simulink model "TST_AFST_DD"  (R2016b)
settings: Solver=FixedStepDiscrete  StartTime=0.0  StopTime=simTime  FixedStep=sampleTime  RelTol=1e-3
values from neighbouring files (symbols this model uses):
  testCase = 1    [initTST_AFST_DD_001.m]    (also in initTST_AFST_DD_002.m = 2; initTST_AFST_DD_003.m = 3; initTST_AFST_DD_004.m = 4)
libraries: simulink x61, UnitTest_Lib x56
(part 1 of 2)
settings Model: Creator=guanxiaoxing  LastModifiedBy=guanxiaoxing
settings DebuggingCC: SignalRangeChecking=error

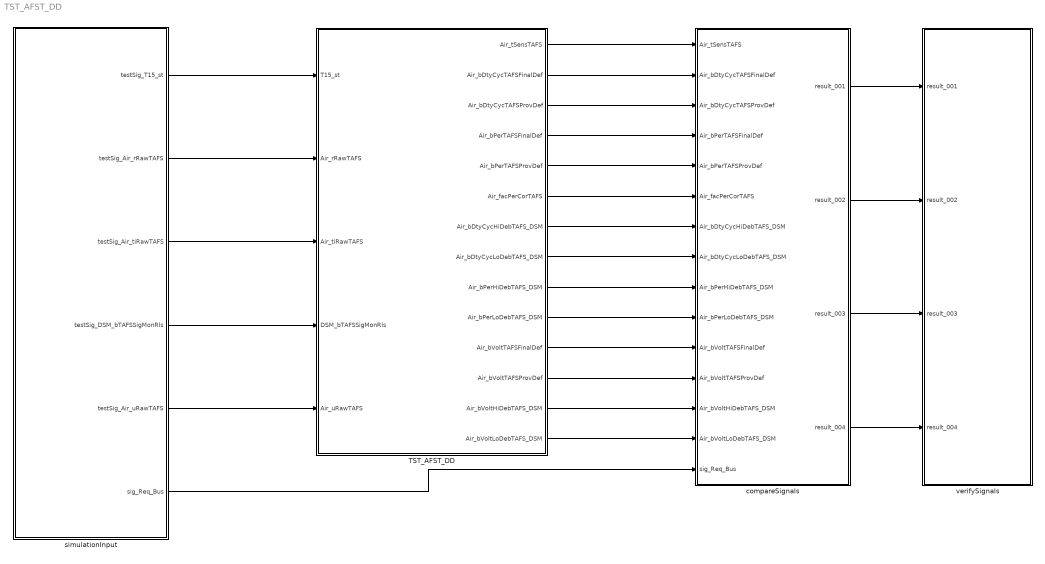
== system TST_AFST_DD ==
  TST_AFST_DD : Subsystem
  compareSignals : Subsystem
  simulationInput : Subsystem
  verifySignals : Subsystem
  wires:
  simulationInput/1(testSig_T15_st) -> TST_AFST_DD/1(T15_st)
  simulationInput/2(testSig_Air_rRawTAFS) -> TST_AFST_DD/2(Air_rRawTAFS)
  simulationInput/3(testSig_Air_tiRawTAFS) -> TST_AFST_DD/3(Air_tiRawTAFS)
  simulationInput/4(testSig_DSM_bTAFSSigMonRls) -> TST_AFST_DD/4(DSM_bTAFSSigMonRls)
  simulationInput/5(testSig_Air_uRawTAFS) -> TST_AFST_DD/5(Air_uRawTAFS)
  TST_AFST_DD/1(Air_tSensTAFS) -> compareSignals/1(Air_tSensTAFS)
  TST_AFST_DD/2(Air_bDtyCycTAFSFinalDef) -> compareSignals/2(Air_bDtyCycTAFSFinalDef)
  TST_AFST_DD/3(Air_bDtyCycTAFSProvDef) -> compareSignals/3(Air_bDtyCycTAFSProvDef)
  TST_AFST_DD/4(Air_bPerTAFSFinalDef) -> compareSignals/4(Air_bPerTAFSFinalDef)
  TST_AFST_DD/5(Air_bPerTAFSProvDef) -> compareSignals/5(Air_bPerTAFSProvDef)
  TST_AFST_DD/6(Air_facPerCorTAFS) -> compareSignals/6(Air_facPerCorTAFS)
  TST_AFST_DD/7(Air_bDtyCycHiDebTAFS_DSM) -> compareSignals/7(Air_bDtyCycHiDebTAFS_DSM)
  TST_AFST_DD/8(Air_bDtyCycLoDebTAFS_DSM) -> compareSignals/8(Air_bDtyCycLoDebTAFS_DSM)
  TST_AFST_DD/9(Air_bPerHiDebTAFS_DSM) -> compareSignals/9(Air_bPerHiDebTAFS_DSM)
  TST_AFST_DD/10(Air_bPerLoDebTAFS_DSM) -> compareSignals/10(Air_bPerLoDebTAFS_DSM)
  TST_AFST_DD/11(Air_bVoltTAFSFinalDef) -> compareSignals/11(Air_bVoltTAFSFinalDef)
  TST_AFST_DD/12(Air_bVoltTAFSProvDef) -> compareSignals/12(Air_bVoltTAFSProvDef)
  TST_AFST_DD/13(Air_bVoltHiDebTAFS_DSM) -> compareSignals/13(Air_bVoltHiDebTAFS_DSM)
  TST_AFST_DD/14(Air_bVoltLoDebTAFS_DSM) -> compareSignals/14(Air_bVoltLoDebTAFS_DSM)
  simulationInput/6(sig_Req_Bus) -> compareSignals/15(sig_Req_Bus)
  compareSignals/1(result_001) -> verifySignals/1(result_001)
  compareSignals/2(result_002) -> verifySignals/2(result_002)
  compareSignals/3(result_003) -> verifySignals/3(result_003)
  compareSignals/4(result_004) -> verifySignals/4(result_004)

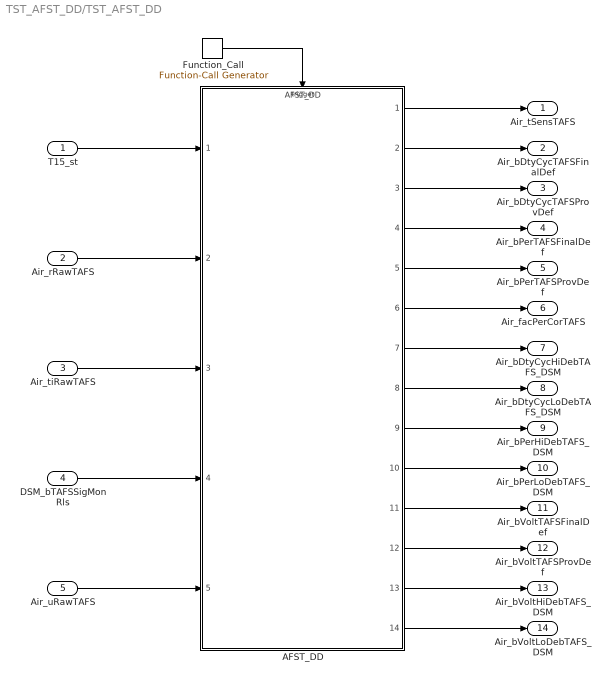
== system TST_AFST_DD/TST_AFST_DD ==
  T15_st : Inport
  Air_rRawTAFS : Inport  Port=2
  Air_tiRawTAFS : Inport  Port=3
  DSM_bTAFSSigMonRls : Inport  Port=4
  Air_uRawTAFS : Inport  Port=5
  AFST_DD : ModelReference  ModelNameDialog=AFST_DD  SimulationMode=Normal  ModelReferenceVersion=1.44  TriggerPortName=function  TriggerPortTriggerType=function-call  TriggerPortStatesWhenEnabling=held
  Function_Call : simulink/Ports & Subsystems/Function-Call Generator  sample_time=sampleTime  numberOfIterations=1
  Air_tSensTAFS : Outport
  Air_bDtyCycTAFSFinalDef : Outport  Port=2
  Air_bDtyCycTAFSProvDef : Outport  Port=3
  Air_bPerTAFSFinalDef : Outport  Port=4
  Air_bPerTAFSProvDef : Outport  Port=5
  Air_facPerCorTAFS : Outport  Port=6
  Air_bDtyCycHiDebTAFS_DSM : Outport  Port=7
  Air_bDtyCycLoDebTAFS_DSM : Outport  Port=8
  Air_bPerHiDebTAFS_DSM : Outport  Port=9
  Air_bPerLoDebTAFS_DSM : Outport  Port=10
  Air_bVoltTAFSFinalDef : Outport  Port=11
  Air_bVoltTAFSProvDef : Outport  Port=12
  Air_bVoltHiDebTAFS_DSM : Outport  Port=13
  Air_bVoltLoDebTAFS_DSM : Outport  Port=14
  wires:
  Function_Call/1 -> AFST_DD/Trigger
  T15_st/1 -> AFST_DD/1
  Air_rRawTAFS/1 -> AFST_DD/2
  Air_tiRawTAFS/1 -> AFST_DD/3
  DSM_bTAFSSigMonRls/1 -> AFST_DD/4
  Air_uRawTAFS/1 -> AFST_DD/5
  AFST_DD/1 -> Air_tSensTAFS/1
  AFST_DD/2 -> Air_bDtyCycTAFSFinalDef/1
  AFST_DD/3 -> Air_bDtyCycTAFSProvDef/1
  AFST_DD/4 -> Air_bPerTAFSFinalDef/1
  AFST_DD/5 -> Air_bPerTAFSProvDef/1
  AFST_DD/6 -> Air_facPerCorTAFS/1
  AFST_DD/7 -> Air_bDtyCycHiDebTAFS_DSM/1
  AFST_DD/8 -> Air_bDtyCycLoDebTAFS_DSM/1
  AFST_DD/9 -> Air_bPerHiDebTAFS_DSM/1
  AFST_DD/10 -> Air_bPerLoDebTAFS_DSM/1
  AFST_DD/11 -> Air_bVoltTAFSFinalDef/1
  AFST_DD/12 -> Air_bVoltTAFSProvDef/1
  AFST_DD/13 -> Air_bVoltHiDebTAFS_DSM/1
  AFST_DD/14 -> Air_bVoltLoDebTAFS_DSM/1

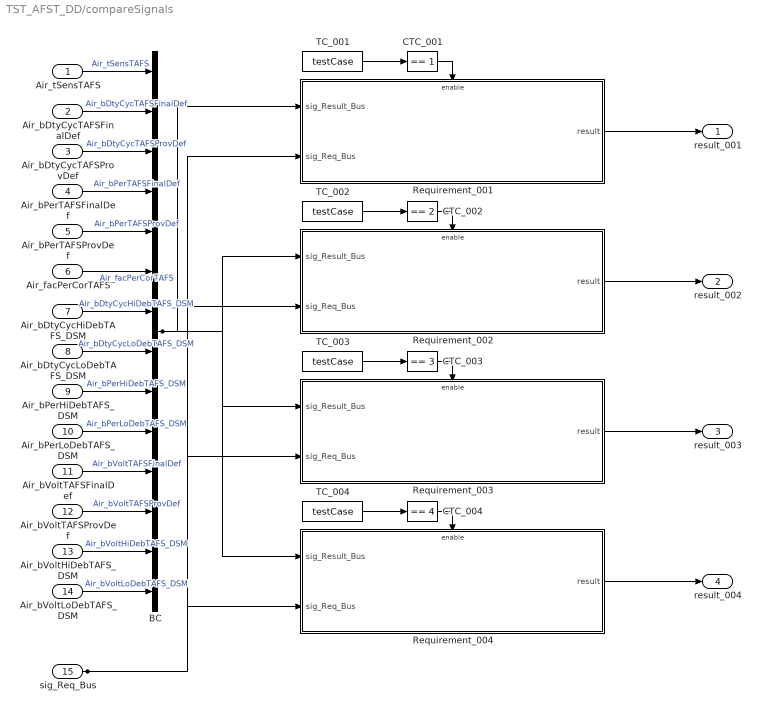
== system TST_AFST_DD/compareSignals ==
  Air_tSensTAFS : Inport
  Air_bDtyCycTAFSFinalDef : Inport  Port=2
  Air_bDtyCycTAFSProvDef : Inport  Port=3
  Air_bPerTAFSFinalDef : Inport  Port=4
  Air_bPerTAFSProvDef : Inport  Port=5
  Air_facPerCorTAFS : Inport  Port=6
  Air_bDtyCycHiDebTAFS_DSM : Inport  Port=7
  Air_bDtyCycLoDebTAFS_DSM : Inport  Port=8
  Air_bPerHiDebTAFS_DSM : Inport  Port=9
  Air_bPerLoDebTAFS_DSM : Inport  Port=10
  Air_bVoltTAFSFinalDef : Inport  Port=11
  Air_bVoltTAFSProvDef : Inport  Port=12
  Air_bVoltHiDebTAFS_DSM : Inport  Port=13
  Air_bVoltLoDebTAFS_DSM : Inport  Port=14
  sig_Req_Bus : Inport  Port=15
  BC : BusCreator  Inputs=14
  CTC_001 : simulink/Logic and Bit Operations/Compare To Constant  relop===  const=1  OutDataTypeStr=boolean
  CTC_002 : simulink/Logic and Bit Operations/Compare To Constant  relop===  const=2  OutDataTypeStr=boolean
  CTC_003 : simulink/Logic and Bit Operations/Compare To Constant  relop===  const=3  OutDataTypeStr=boolean
  CTC_004 : simulink/Logic and Bit Operations/Compare To Constant  relop===  const=4  OutDataTypeStr=boolean
  Requirement_001 : Subsystem
  Requirement_002 : Subsystem
  Requirement_003 : Subsystem
  Requirement_004 : Subsystem
  TC_001 : Constant  Value=testCase
  TC_002 : Constant  Value=testCase
  TC_003 : Constant  Value=testCase
  TC_004 : Constant  Value=testCase
  result_001 : Outport
  result_002 : Outport  Port=2
  result_003 : Outport  Port=3
  result_004 : Outport  Port=4
  wires:
  Air_tSensTAFS/1 -> BC/1  "Air_tSensTAFS"
  Air_bDtyCycTAFSFinalDef/1 -> BC/2  "Air_bDtyCycTAFSFinalDef"
  Air_bDtyCycTAFSProvDef/1 -> BC/3  "Air_bDtyCycTAFSProvDef"
  Air_bPerTAFSFinalDef/1 -> BC/4  "Air_bPerTAFSFinalDef"
  Air_bPerTAFSProvDef/1 -> BC/5  "Air_bPerTAFSProvDef"
  Air_facPerCorTAFS/1 -> BC/6  "Air_facPerCorTAFS"
  Air_bDtyCycHiDebTAFS_DSM/1 -> BC/7  "Air_bDtyCycHiDebTAFS_DSM"
  Air_bDtyCycLoDebTAFS_DSM/1 -> BC/8  "Air_bDtyCycLoDebTAFS_DSM"
  Air_bPerHiDebTAFS_DSM/1 -> BC/9  "Air_bPerHiDebTAFS_DSM"
  Air_bPerLoDebTAFS_DSM/1 -> BC/10  "Air_bPerLoDebTAFS_DSM"
  Air_bVoltTAFSFinalDef/1 -> BC/11  "Air_bVoltTAFSFinalDef"
  Air_bVoltTAFSProvDef/1 -> BC/12  "Air_bVoltTAFSProvDef"
  Air_bVoltHiDebTAFS_DSM/1 -> BC/13  "Air_bVoltHiDebTAFS_DSM"
  Air_bVoltLoDebTAFS_DSM/1 -> BC/14  "Air_bVoltLoDebTAFS_DSM"
  TC_001/1 -> CTC_001/1
  CTC_001/1 -> Requirement_001/Enable
  sig_Req_Bus/1 -> Requirement_001/2(sig_Req_Bus), Requirement_002/2(sig_Req_Bus), Requirement_003/2(sig_Req_Bus), Requirement_004/2(sig_Req_Bus)
  BC/1 -> Requirement_001/1(sig_Result_Bus), Requirement_002/1(sig_Result_Bus), Requirement_003/1(sig_Result_Bus), Requirement_004/1(sig_Result_Bus)
  Requirement_001/1(result) -> result_001/1
  TC_002/1 -> CTC_002/1
  CTC_002/1 -> Requirement_002/Enable
  Requirement_002/1(result) -> result_002/1
  TC_003/1 -> CTC_003/1
  CTC_003/1 -> Requirement_003/Enable
  Requirement_003/1(result) -> result_003/1
  TC_004/1 -> CTC_004/1
  CTC_004/1 -> Requirement_004/Enable
  Requirement_004/1(result) -> result_004/1

== system TST_AFST_DD/simulationInput ==
  BS : BusSelector  OutputSignals=testSig_T15_st,testSig_Air_rRawTAFS,testSig_Air_tiRawTAFS,testSig_DSM_bTAFSSigMonRls,testSig_Air_uRawTAFS
  MPSw : MultiPortSwitch  Inputs=4  SaturateOnIntegerOverflow=on  InputSameDT=on
  TestCase : Constant  Value=testCase
  testSignals_R001 : Subsystem
  testSignals_R002 : Subsystem
  testSignals_R003 : Subsystem
  testSignals_R004 : Subsystem
  testSig_T15_st : Outport
  testSig_Air_rRawTAFS : Outport  Port=2
  testSig_Air_tiRawTAFS : Outport  Port=3
  testSig_DSM_bTAFSSigMonRls : Outport  Port=4
  testSig_Air_uRawTAFS : Outport  Port=5
  sig_Req_Bus : Outport  Port=6
  wires:
  BS/1 -> testSig_T15_st/1  "<testSig_T15_st>"
  BS/2 -> testSig_Air_rRawTAFS/1  "<testSig_Air_rRawTAFS>"
  BS/3 -> testSig_Air_tiRawTAFS/1  "<testSig_Air_tiRawTAFS>"
  BS/4 -> testSig_DSM_bTAFSSigMonRls/1  "<testSig_DSM_bTAFSSigMonRls>"
  BS/5 -> testSig_Air_uRawTAFS/1  "<testSig_Air_uRawTAFS>"
  MPSw/1 -> BS/1, sig_Req_Bus/1
  TestCase/1 -> MPSw/1
  testSignals_R001/1(testSignals) -> MPSw/2
  testSignals_R002/1(testSignals) -> MPSw/3
  testSignals_R003/1(testSignals) -> MPSw/4
  testSignals_R004/1(testSignals) -> MPSw/5

== system TST_AFST_DD/verifySignals ==
  result_001 : Inport
  result_002 : Inport  Port=2
  result_003 : Inport  Port=3
  result_004 : Inport  Port=4
  Assertion_001 : Assertion  Enabled=off
  Assertion_002 : Assertion  Enabled=off
  Assertion_003 : Assertion  Enabled=off
  Assertion_004 : Assertion  Enabled=off
  wires:
  result_001/1 -> Assertion_001/1
  result_002/1 -> Assertion_002/1
  result_003/1 -> Assertion_003/1
  result_004/1 -> Assertion_004/1

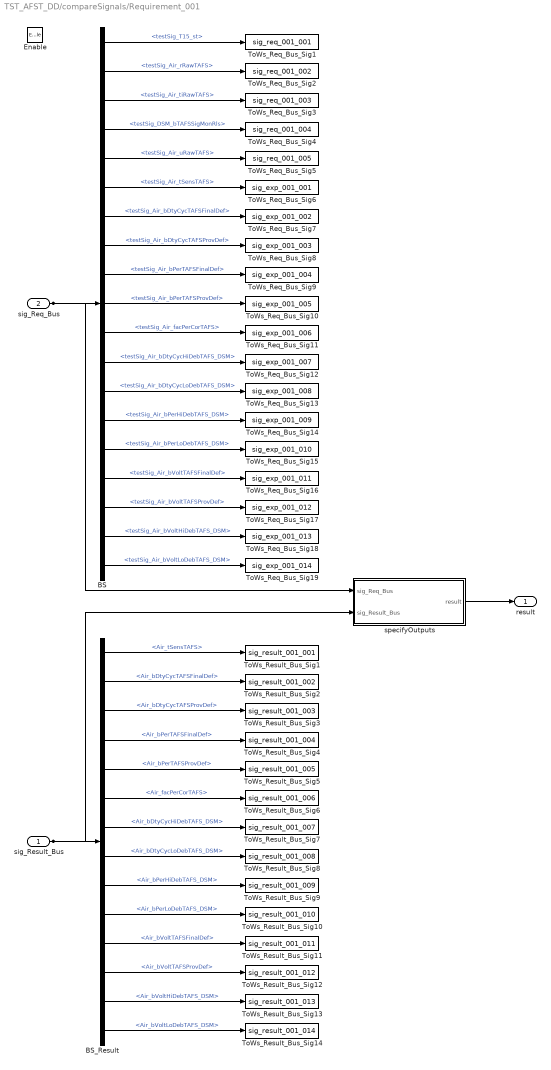
== system TST_AFST_DD/compareSignals/Requirement_001 ==
  sig_Result_Bus : Inport
  sig_Req_Bus : Inport  Port=2
  Enable : EnablePort
  BS : BusSelector  OutputSignals=testSig_T15_st,testSig_Air_rRawTAFS,testSig_Air_tiRawTAFS,testSig_DSM_bTAFSSigMonRls,testSig_Air_uRawTAFS,testSig_Air_tSensTAFS,testSig_Air_bDtyCycTAFSFinalDef,testSig_Air_bDtyCycTAFSProvDef,testSig_Air_bPerTAFSFinalDef,testSig_Air_bPerTAFSProvDef,testSig_Air_facPerCorTAFS,testSig_Air_bDtyCycHiDebTAFS_DSM,testSig_Air_bDtyCycLoDebTAFS_DSM,testSig_Air_bPerHiDebTAFS_DSM,testSig_Air_bPerLoDebTAFS_DSM,testSig_Air_bVoltTAFSFinalDef,testSig_Air_bVoltTAFSProvDef,testSig_Air_bVoltHiDebTAFS_DSM,testSig_Air_bVoltLoDebTAFS_DSM
  BS_Result : BusSelector  OutputSignals=Air_tSensTAFS,Air_bDtyCycTAFSFinalDef,Air_bDtyCycTAFSProvDef,Air_bPerTAFSFinalDef,Air_bPerTAFSProvDef,Air_facPerCorTAFS,Air_bDtyCycHiDebTAFS_DSM,Air_bDtyCycLoDebTAFS_DSM,Air_bPerHiDebTAFS_DSM,Air_bPerLoDebTAFS_DSM,Air_bVoltTAFSFinalDef,Air_bVoltTAFSProvDef,Air_bVoltHiDebTAFS_DSM,Air_bVoltLoDebTAFS_DSM
  ToWs_Req_Bus_Sig1 : ToWorkspace  VariableName=sig_req_001_001  SaveFormat=Structure With Time
  ToWs_Req_Bus_Sig10 : ToWorkspace  VariableName=sig_exp_001_005  SaveFormat=Structure With Time
  ToWs_Req_Bus_Sig11 : ToWorkspace  VariableName=sig_exp_001_006  SaveFormat=Structure With Time
  ToWs_Req_Bus_Sig12 : ToWorkspace  VariableName=sig_exp_001_007  SaveFormat=Structure With Time
  ToWs_Req_Bus_Sig13 : ToWorkspace  VariableName=sig_exp_001_008  SaveFormat=Structure With Time
  ToWs_Req_Bus_Sig14 : ToWorkspace  VariableName=sig_exp_001_009  SaveFormat=Structure With Time
  ToWs_Req_Bus_Sig15 : ToWorkspace  VariableName=sig_exp_001_010  SaveFormat=Structure With Time
  ToWs_Req_Bus_Sig16 : ToWorkspace  VariableName=sig_exp_001_011  SaveFormat=Structure With Time
  ToWs_Req_Bus_Sig17 : ToWorkspace  VariableName=sig_exp_001_012  SaveFormat=Structure With Time
  ToWs_Req_Bus_Sig18 : ToWorkspace  VariableName=sig_exp_001_013  SaveFormat=Structure With Time
  ToWs_Req_Bus_Sig19 : ToWorkspace  VariableName=sig_exp_001_014  SaveFormat=Structure With Time
  ToWs_Req_Bus_Sig2 : ToWorkspace  VariableName=sig_req_001_002  SaveFormat=Structure With Time
  ToWs_Req_Bus_Sig3 : ToWorkspace  VariableName=sig_req_001_003  SaveFormat=Structure With Time
  ToWs_Req_Bus_Sig4 : ToWorkspace  VariableName=sig_req_001_004  SaveFormat=Structure With Time
  ToWs_Req_Bus_Sig5 : ToWorkspace  VariableName=sig_req_001_005  SaveFormat=Structure With Time
  ToWs_Req_Bus_Sig6 : ToWorkspace  VariableName=sig_exp_001_001  SaveFormat=Structure With Time
  ToWs_Req_Bus_Sig7 : ToWorkspace  VariableName=sig_exp_001_002  SaveFormat=Structure With Time
  ToWs_Req_Bus_Sig8 : ToWorkspace  VariableName=sig_exp_001_003  SaveFormat=Structure With Time
  ToWs_Req_Bus_Sig9 : ToWorkspace  VariableName=sig_exp_001_004  SaveFormat=Structure With Time
  ToWs_Result_Bus_Sig1 : ToWorkspace  VariableName=sig_result_001_001  SaveFormat=Structure With Time
  ToWs_Result_Bus_Sig10 : ToWorkspace  VariableName=sig_result_001_010  SaveFormat=Structure With Time
  ToWs_Result_Bus_Sig11 : ToWorkspace  VariableName=sig_result_001_011  SaveFormat=Structure With Time
  ToWs_Result_Bus_Sig12 : ToWorkspace  VariableName=sig_result_001_012  SaveFormat=Structure With Time
  ToWs_Result_Bus_Sig13 : ToWorkspace  VariableName=sig_result_001_013  SaveFormat=Structure With Time
  ToWs_Result_Bus_Sig14 : ToWorkspace  VariableName=sig_result_001_014  SaveFormat=Structure With Time
  ToWs_Result_Bus_Sig2 : ToWorkspace  VariableName=sig_result_001_002  SaveFormat=Structure With Time
  ToWs_Result_Bus_Sig3 : ToWorkspace  VariableName=sig_result_001_003  SaveFormat=Structure With Time
  ToWs_Result_Bus_Sig4 : ToWorkspace  VariableName=sig_result_001_004  SaveFormat=Structure With Time
  ToWs_Result_Bus_Sig5 : ToWorkspace  VariableName=sig_result_001_005  SaveFormat=Structure With Time
  ToWs_Result_Bus_Sig6 : ToWorkspace  VariableName=sig_result_001_006  SaveFormat=Structure With Time
  ToWs_Result_Bus_Sig7 : ToWorkspace  VariableName=sig_result_001_007  SaveFormat=Structure With Time
  ToWs_Result_Bus_Sig8 : ToWorkspace  VariableName=sig_result_001_008  SaveFormat=Structure With Time
  ToWs_Result_Bus_Sig9 : ToWorkspace  VariableName=sig_result_001_009  SaveFormat=Structure With Time
  specifyOutputs : Subsystem
  result : Outport
  wires:
  sig_Req_Bus/1 -> BS/1, specifyOutputs/1(sig_Req_Bus)
  BS/1 -> ToWs_Req_Bus_Sig1/1  "<testSig_T15_st>"
  BS/2 -> ToWs_Req_Bus_Sig2/1  "<testSig_Air_rRawTAFS>"
  BS/3 -> ToWs_Req_Bus_Sig3/1  "<testSig_Air_tiRawTAFS>"
  BS/4 -> ToWs_Req_Bus_Sig4/1  "<testSig_DSM_bTAFSSigMonRls>"
  BS/5 -> ToWs_Req_Bus_Sig5/1  "<testSig_Air_uRawTAFS>"
  BS/6 -> ToWs_Req_Bus_Sig6/1  "<testSig_Air_tSensTAFS>"
  BS/7 -> ToWs_Req_Bus_Sig7/1  "<testSig_Air_bDtyCycTAFSFinalDef>"
  BS/8 -> ToWs_Req_Bus_Sig8/1  "<testSig_Air_bDtyCycTAFSProvDef>"
  BS/9 -> ToWs_Req_Bus_Sig9/1  "<testSig_Air_bPerTAFSFinalDef>"
  BS/10 -> ToWs_Req_Bus_Sig10/1  "<testSig_Air_bPerTAFSProvDef>"
  BS/11 -> ToWs_Req_Bus_Sig11/1  "<testSig_Air_facPerCorTAFS>"
  BS/12 -> ToWs_Req_Bus_Sig12/1  "<testSig_Air_bDtyCycHiDebTAFS_DSM>"
  BS/13 -> ToWs_Req_Bus_Sig13/1  "<testSig_Air_bDtyCycLoDebTAFS_DSM>"
  BS/14 -> ToWs_Req_Bus_Sig14/1  "<testSig_Air_bPerHiDebTAFS_DSM>"
  BS/15 -> ToWs_Req_Bus_Sig15/1  "<testSig_Air_bPerLoDebTAFS_DSM>"
  BS/16 -> ToWs_Req_Bus_Sig16/1  "<testSig_Air_bVoltTAFSFinalDef>"
  BS/17 -> ToWs_Req_Bus_Sig17/1  "<testSig_Air_bVoltTAFSProvDef>"
  BS/18 -> ToWs_Req_Bus_Sig18/1  "<testSig_Air_bVoltHiDebTAFS_DSM>"
  BS/19 -> ToWs_Req_Bus_Sig19/1  "<testSig_Air_bVoltLoDebTAFS_DSM>"
  sig_Result_Bus/1 -> BS_Result/1, specifyOutputs/2(sig_Result_Bus)
  BS_Result/1 -> ToWs_Result_Bus_Sig1/1  "<Air_tSensTAFS>"
  BS_Result/2 -> ToWs_Result_Bus_Sig2/1  "<Air_bDtyCycTAFSFinalDef>"
  BS_Result/3 -> ToWs_Result_Bus_Sig3/1  "<Air_bDtyCycTAFSProvDef>"
  BS_Result/4 -> ToWs_Result_Bus_Sig4/1  "<Air_bPerTAFSFinalDef>"
  BS_Result/5 -> ToWs_Result_Bus_Sig5/1  "<Air_bPerTAFSProvDef>"
  BS_Result/6 -> ToWs_Result_Bus_Sig6/1  "<Air_facPerCorTAFS>"
  BS_Result/7 -> ToWs_Result_Bus_Sig7/1  "<Air_bDtyCycHiDebTAFS_DSM>"
  BS_Result/8 -> ToWs_Result_Bus_Sig8/1  "<Air_bDtyCycLoDebTAFS_DSM>"
  BS_Result/9 -> ToWs_Result_Bus_Sig9/1  "<Air_bPerHiDebTAFS_DSM>"
  BS_Result/10 -> ToWs_Result_Bus_Sig10/1  "<Air_bPerLoDebTAFS_DSM>"
  BS_Result/11 -> ToWs_Result_Bus_Sig11/1  "<Air_bVoltTAFSFinalDef>"
  BS_Result/12 -> ToWs_Result_Bus_Sig12/1  "<Air_bVoltTAFSProvDef>"
  BS_Result/13 -> ToWs_Result_Bus_Sig13/1  "<Air_bVoltHiDebTAFS_DSM>"
  BS_Result/14 -> ToWs_Result_Bus_Sig14/1  "<Air_bVoltLoDebTAFS_DSM>"
  specifyOutputs/1(result) -> result/1

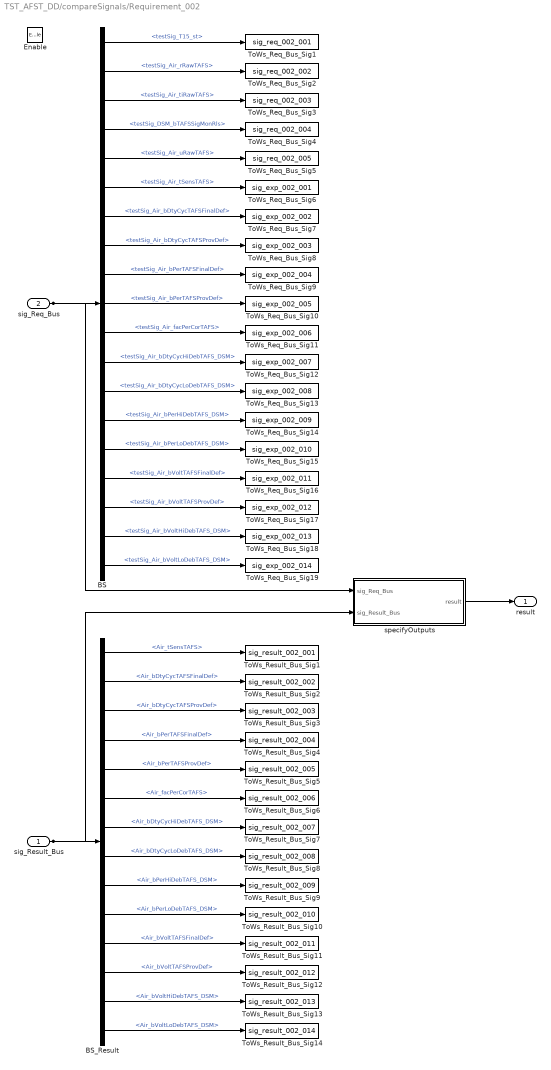
== system TST_AFST_DD/compareSignals/Requirement_002 ==
  sig_Result_Bus : Inport
  sig_Req_Bus : Inport  Port=2
  Enable : EnablePort
  BS : BusSelector  OutputSignals=testSig_T15_st,testSig_Air_rRawTAFS,testSig_Air_tiRawTAFS,testSig_DSM_bTAFSSigMonRls,testSig_Air_uRawTAFS,testSig_Air_tSensTAFS,testSig_Air_bDtyCycTAFSFinalDef,testSig_Air_bDtyCycTAFSProvDef,testSig_Air_bPerTAFSFinalDef,testSig_Air_bPerTAFSProvDef,testSig_Air_facPerCorTAFS,testSig_Air_bDtyCycHiDebTAFS_DSM,testSig_Air_bDtyCycLoDebTAFS_DSM,testSig_Air_bPerHiDebTAFS_DSM,testSig_Air_bPerLoDebTAFS_DSM,testSig_Air_bVoltTAFSFinalDef,testSig_Air_bVoltTAFSProvDef,testSig_Air_bVoltHiDebTAFS_DSM,testSig_Air_bVoltLoDebTAFS_DSM
  BS_Result : BusSelector  OutputSignals=Air_tSensTAFS,Air_bDtyCycTAFSFinalDef,Air_bDtyCycTAFSProvDef,Air_bPerTAFSFinalDef,Air_bPerTAFSProvDef,Air_facPerCorTAFS,Air_bDtyCycHiDebTAFS_DSM,Air_bDtyCycLoDebTAFS_DSM,Air_bPerHiDebTAFS_DSM,Air_bPerLoDebTAFS_DSM,Air_bVoltTAFSFinalDef,Air_bVoltTAFSProvDef,Air_bVoltHiDebTAFS_DSM,Air_bVoltLoDebTAFS_DSM
  ToWs_Req_Bus_Sig1 : ToWorkspace  VariableName=sig_req_002_001  SaveFormat=Structure With Time
  ToWs_Req_Bus_Sig10 : ToWorkspace  VariableName=sig_exp_002_005  SaveFormat=Structure With Time
  ToWs_Req_Bus_Sig11 : ToWorkspace  VariableName=sig_exp_002_006  SaveFormat=Structure With Time
  ToWs_Req_Bus_Sig12 : ToWorkspace  VariableName=sig_exp_002_007  SaveFormat=Structure With Time
  ToWs_Req_Bus_Sig13 : ToWorkspace  VariableName=sig_exp_002_008  SaveFormat=Structure With Time
  ToWs_Req_Bus_Sig14 : ToWorkspace  VariableName=sig_exp_002_009  SaveFormat=Structure With Time
  ToWs_Req_Bus_Sig15 : ToWorkspace  VariableName=sig_exp_002_010  SaveFormat=Structure With Time
  ToWs_Req_Bus_Sig16 : ToWorkspace  VariableName=sig_exp_002_011  SaveFormat=Structure With Time
  ToWs_Req_Bus_Sig17 : ToWorkspace  VariableName=sig_exp_002_012  SaveFormat=Structure With Time
  ToWs_Req_Bus_Sig18 : ToWorkspace  VariableName=sig_exp_002_013  SaveFormat=Structure With Time
  ToWs_Req_Bus_Sig19 : ToWorkspace  VariableName=sig_exp_002_014  SaveFormat=Structure With Time
  ToWs_Req_Bus_Sig2 : ToWorkspace  VariableName=sig_req_002_002  SaveFormat=Structure With Time
  ToWs_Req_Bus_Sig3 : ToWorkspace  VariableName=sig_req_002_003  SaveFormat=Structure With Time
  ToWs_Req_Bus_Sig4 : ToWorkspace  VariableName=sig_req_002_004  SaveFormat=Structure With Time
  ToWs_Req_Bus_Sig5 : ToWorkspace  VariableName=sig_req_002_005  SaveFormat=Structure With Time
  ToWs_Req_Bus_Sig6 : ToWorkspace  VariableName=sig_exp_002_001  SaveFormat=Structure With Time
  ToWs_Req_Bus_Sig7 : ToWorkspace  VariableName=sig_exp_002_002  SaveFormat=Structure With Time
  ToWs_Req_Bus_Sig8 : ToWorkspace  VariableName=sig_exp_002_003  SaveFormat=Structure With Time
  ToWs_Req_Bus_Sig9 : ToWorkspace  VariableName=sig_exp_002_004  SaveFormat=Structure With Time
  ToWs_Result_Bus_Sig1 : ToWorkspace  VariableName=sig_result_002_001  SaveFormat=Structure With Time
  ToWs_Result_Bus_Sig10 : ToWorkspace  VariableName=sig_result_002_010  SaveFormat=Structure With Time
  ToWs_Result_Bus_Sig11 : ToWorkspace  VariableName=sig_result_002_011  SaveFormat=Structure With Time
  ToWs_Result_Bus_Sig12 : ToWorkspace  VariableName=sig_result_002_012  SaveFormat=Structure With Time
  ToWs_Result_Bus_Sig13 : ToWorkspace  VariableName=sig_result_002_013  SaveFormat=Structure With Time
  ToWs_Result_Bus_Sig14 : ToWorkspace  VariableName=sig_result_002_014  SaveFormat=Structure With Time
  ToWs_Result_Bus_Sig2 : ToWorkspace  VariableName=sig_result_002_002  SaveFormat=Structure With Time
  ToWs_Result_Bus_Sig3 : ToWorkspace  VariableName=sig_result_002_003  SaveFormat=Structure With Time
  ToWs_Result_Bus_Sig4 : ToWorkspace  VariableName=sig_result_002_004  SaveFormat=Structure With Time
  ToWs_Result_Bus_Sig5 : ToWorkspace  VariableName=sig_result_002_005  SaveFormat=Structure With Time
  ToWs_Result_Bus_Sig6 : ToWorkspace  VariableName=sig_result_002_006  SaveFormat=Structure With Time
  ToWs_Result_Bus_Sig7 : ToWorkspace  VariableName=sig_result_002_007  SaveFormat=Structure With Time
  ToWs_Result_Bus_Sig8 : ToWorkspace  VariableName=sig_result_002_008  SaveFormat=Structure With Time
  ToWs_Result_Bus_Sig9 : ToWorkspace  VariableName=sig_result_002_009  SaveFormat=Structure With Time
  specifyOutputs : Subsystem
  result : Outport
  wires:
  sig_Req_Bus/1 -> BS/1, specifyOutputs/1(sig_Req_Bus)
  BS/1 -> ToWs_Req_Bus_Sig1/1  "<testSig_T15_st>"
  BS/2 -> ToWs_Req_Bus_Sig2/1  "<testSig_Air_rRawTAFS>"
  BS/3 -> ToWs_Req_Bus_Sig3/1  "<testSig_Air_tiRawTAFS>"
  BS/4 -> ToWs_Req_Bus_Sig4/1  "<testSig_DSM_bTAFSSigMonRls>"
  BS/5 -> ToWs_Req_Bus_Sig5/1  "<testSig_Air_uRawTAFS>"
  BS/6 -> ToWs_Req_Bus_Sig6/1  "<testSig_Air_tSensTAFS>"
  BS/7 -> ToWs_Req_Bus_Sig7/1  "<testSig_Air_bDtyCycTAFSFinalDef>"
  BS/8 -> ToWs_Req_Bus_Sig8/1  "<testSig_Air_bDtyCycTAFSProvDef>"
  BS/9 -> ToWs_Req_Bus_Sig9/1  "<testSig_Air_bPerTAFSFinalDef>"
  BS/10 -> ToWs_Req_Bus_Sig10/1  "<testSig_Air_bPerTAFSProvDef>"
  BS/11 -> ToWs_Req_Bus_Sig11/1  "<testSig_Air_facPerCorTAFS>"
  BS/12 -> ToWs_Req_Bus_Sig12/1  "<testSig_Air_bDtyCycHiDebTAFS_DSM>"
  BS/13 -> ToWs_Req_Bus_Sig13/1  "<testSig_Air_bDtyCycLoDebTAFS_DSM>"
  BS/14 -> ToWs_Req_Bus_Sig14/1  "<testSig_Air_bPerHiDebTAFS_DSM>"
  BS/15 -> ToWs_Req_Bus_Sig15/1  "<testSig_Air_bPerLoDebTAFS_DSM>"
  BS/16 -> ToWs_Req_Bus_Sig16/1  "<testSig_Air_bVoltTAFSFinalDef>"
  BS/17 -> ToWs_Req_Bus_Sig17/1  "<testSig_Air_bVoltTAFSProvDef>"
  BS/18 -> ToWs_Req_Bus_Sig18/1  "<testSig_Air_bVoltHiDebTAFS_DSM>"
  BS/19 -> ToWs_Req_Bus_Sig19/1  "<testSig_Air_bVoltLoDebTAFS_DSM>"
  sig_Result_Bus/1 -> BS_Result/1, specifyOutputs/2(sig_Result_Bus)
  BS_Result/1 -> ToWs_Result_Bus_Sig1/1  "<Air_tSensTAFS>"
  BS_Result/2 -> ToWs_Result_Bus_Sig2/1  "<Air_bDtyCycTAFSFinalDef>"
  BS_Result/3 -> ToWs_Result_Bus_Sig3/1  "<Air_bDtyCycTAFSProvDef>"
  BS_Result/4 -> ToWs_Result_Bus_Sig4/1  "<Air_bPerTAFSFinalDef>"
  BS_Result/5 -> ToWs_Result_Bus_Sig5/1  "<Air_bPerTAFSProvDef>"
  BS_Result/6 -> ToWs_Result_Bus_Sig6/1  "<Air_facPerCorTAFS>"
  BS_Result/7 -> ToWs_Result_Bus_Sig7/1  "<Air_bDtyCycHiDebTAFS_DSM>"
  BS_Result/8 -> ToWs_Result_Bus_Sig8/1  "<Air_bDtyCycLoDebTAFS_DSM>"
  BS_Result/9 -> ToWs_Result_Bus_Sig9/1  "<Air_bPerHiDebTAFS_DSM>"
  BS_Result/10 -> ToWs_Result_Bus_Sig10/1  "<Air_bPerLoDebTAFS_DSM>"
  BS_Result/11 -> ToWs_Result_Bus_Sig11/1  "<Air_bVoltTAFSFinalDef>"
  BS_Result/12 -> ToWs_Result_Bus_Sig12/1  "<Air_bVoltTAFSProvDef>"
  BS_Result/13 -> ToWs_Result_Bus_Sig13/1  "<Air_bVoltHiDebTAFS_DSM>"
  BS_Result/14 -> ToWs_Result_Bus_Sig14/1  "<Air_bVoltLoDebTAFS_DSM>"
  specifyOutputs/1(result) -> result/1

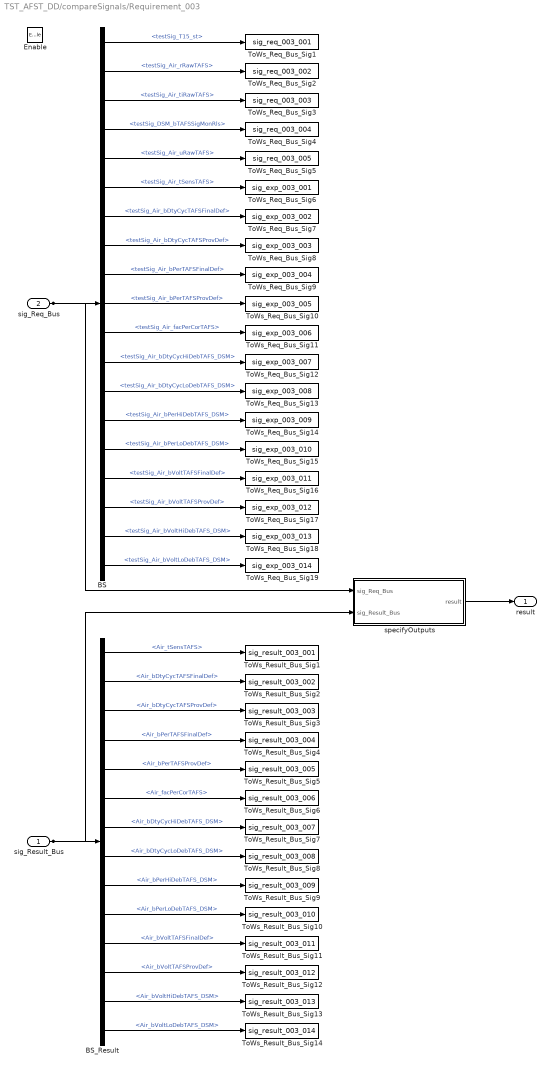
== system TST_AFST_DD/compareSignals/Requirement_003 ==
  sig_Result_Bus : Inport
  sig_Req_Bus : Inport  Port=2
  Enable : EnablePort
  BS : BusSelector  OutputSignals=testSig_T15_st,testSig_Air_rRawTAFS,testSig_Air_tiRawTAFS,testSig_DSM_bTAFSSigMonRls,testSig_Air_uRawTAFS,testSig_Air_tSensTAFS,testSig_Air_bDtyCycTAFSFinalDef,testSig_Air_bDtyCycTAFSProvDef,testSig_Air_bPerTAFSFinalDef,testSig_Air_bPerTAFSProvDef,testSig_Air_facPerCorTAFS,testSig_Air_bDtyCycHiDebTAFS_DSM,testSig_Air_bDtyCycLoDebTAFS_DSM,testSig_Air_bPerHiDebTAFS_DSM,testSig_Air_bPerLoDebTAFS_DSM,testSig_Air_bVoltTAFSFinalDef,testSig_Air_bVoltTAFSProvDef,testSig_Air_bVoltHiDebTAFS_DSM,testSig_Air_bVoltLoDebTAFS_DSM
  BS_Result : BusSelector  OutputSignals=Air_tSensTAFS,Air_bDtyCycTAFSFinalDef,Air_bDtyCycTAFSProvDef,Air_bPerTAFSFinalDef,Air_bPerTAFSProvDef,Air_facPerCorTAFS,Air_bDtyCycHiDebTAFS_DSM,Air_bDtyCycLoDebTAFS_DSM,Air_bPerHiDebTAFS_DSM,Air_bPerLoDebTAFS_DSM,Air_bVoltTAFSFinalDef,Air_bVoltTAFSProvDef,Air_bVoltHiDebTAFS_DSM,Air_bVoltLoDebTAFS_DSM
  ToWs_Req_Bus_Sig1 : ToWorkspace  VariableName=sig_req_003_001  SaveFormat=Structure With Time
  ToWs_Req_Bus_Sig10 : ToWorkspace  VariableName=sig_exp_003_005  SaveFormat=Structure With Time
  ToWs_Req_Bus_Sig11 : ToWorkspace  VariableName=sig_exp_003_006  SaveFormat=Structure With Time
  ToWs_Req_Bus_Sig12 : ToWorkspace  VariableName=sig_exp_003_007  SaveFormat=Structure With Time
  ToWs_Req_Bus_Sig13 : ToWorkspace  VariableName=sig_exp_003_008  SaveFormat=Structure With Time
  ToWs_Req_Bus_Sig14 : ToWorkspace  VariableName=sig_exp_003_009  SaveFormat=Structure With Time
  ToWs_Req_Bus_Sig15 : ToWorkspace  VariableName=sig_exp_003_010  SaveFormat=Structure With Time
  ToWs_Req_Bus_Sig16 : ToWorkspace  VariableName=sig_exp_003_011  SaveFormat=Structure With Time
  ToWs_Req_Bus_Sig17 : ToWorkspace  VariableName=sig_exp_003_012  SaveFormat=Structure With Time
  ToWs_Req_Bus_Sig18 : ToWorkspace  VariableName=sig_exp_003_013  SaveFormat=Structure With Time
  ToWs_Req_Bus_Sig19 : ToWorkspace  VariableName=sig_exp_003_014  SaveFormat=Structure With Time
  ToWs_Req_Bus_Sig2 : ToWorkspace  VariableName=sig_req_003_002  SaveFormat=Structure With Time
  ToWs_Req_Bus_Sig3 : ToWorkspace  VariableName=sig_req_003_003  SaveFormat=Structure With Time
  ToWs_Req_Bus_Sig4 : ToWorkspace  VariableName=sig_req_003_004  SaveFormat=Structure With Time
  ToWs_Req_Bus_Sig5 : ToWorkspace  VariableName=sig_req_003_005  SaveFormat=Structure With Time
  ToWs_Req_Bus_Sig6 : ToWorkspace  VariableName=sig_exp_003_001  SaveFormat=Structure With Time
  ToWs_Req_Bus_Sig7 : ToWorkspace  VariableName=sig_exp_003_002  SaveFormat=Structure With Time
  ToWs_Req_Bus_Sig8 : ToWorkspace  VariableName=sig_exp_003_003  SaveFormat=Structure With Time
  ToWs_Req_Bus_Sig9 : ToWorkspace  VariableName=sig_exp_003_004  SaveFormat=Structure With Time
  ToWs_Result_Bus_Sig1 : ToWorkspace  VariableName=sig_result_003_001  SaveFormat=Structure With Time
  ToWs_Result_Bus_Sig10 : ToWorkspace  VariableName=sig_result_003_010  SaveFormat=Structure With Time
  ToWs_Result_Bus_Sig11 : ToWorkspace  VariableName=sig_result_003_011  SaveFormat=Structure With Time
  ToWs_Result_Bus_Sig12 : ToWorkspace  VariableName=sig_result_003_012  SaveFormat=Structure With Time
  ToWs_Result_Bus_Sig13 : ToWorkspace  VariableName=sig_result_003_013  SaveFormat=Structure With Time
  ToWs_Result_Bus_Sig14 : ToWorkspace  VariableName=sig_result_003_014  SaveFormat=Structure With Time
  ToWs_Result_Bus_Sig2 : ToWorkspace  VariableName=sig_result_003_002  SaveFormat=Structure With Time
  ToWs_Result_Bus_Sig3 : ToWorkspace  VariableName=sig_result_003_003  SaveFormat=Structure With Time
  ToWs_Result_Bus_Sig4 : ToWorkspace  VariableName=sig_result_003_004  SaveFormat=Structure With Time
  ToWs_Result_Bus_Sig5 : ToWorkspace  VariableName=sig_result_003_005  SaveFormat=Structure With Time
  ToWs_Result_Bus_Sig6 : ToWorkspace  VariableName=sig_result_003_006  SaveFormat=Structure With Time
  ToWs_Result_Bus_Sig7 : ToWorkspace  VariableName=sig_result_003_007  SaveFormat=Structure With Time
  ToWs_Result_Bus_Sig8 : ToWorkspace  VariableName=sig_result_003_008  SaveFormat=Structure With Time
  ToWs_Result_Bus_Sig9 : ToWorkspace  VariableName=sig_result_003_009  SaveFormat=Structure With Time
  specifyOutputs : Subsystem
  result : Outport
  wires:
  sig_Req_Bus/1 -> BS/1, specifyOutputs/1(sig_Req_Bus)
  BS/1 -> ToWs_Req_Bus_Sig1/1  "<testSig_T15_st>"
  BS/2 -> ToWs_Req_Bus_Sig2/1  "<testSig_Air_rRawTAFS>"
  BS/3 -> ToWs_Req_Bus_Sig3/1  "<testSig_Air_tiRawTAFS>"
  BS/4 -> ToWs_Req_Bus_Sig4/1  "<testSig_DSM_bTAFSSigMonRls>"
  BS/5 -> ToWs_Req_Bus_Sig5/1  "<testSig_Air_uRawTAFS>"
  BS/6 -> ToWs_Req_Bus_Sig6/1  "<testSig_Air_tSensTAFS>"
  BS/7 -> ToWs_Req_Bus_Sig7/1  "<testSig_Air_bDtyCycTAFSFinalDef>"
  BS/8 -> ToWs_Req_Bus_Sig8/1  "<testSig_Air_bDtyCycTAFSProvDef>"
  BS/9 -> ToWs_Req_Bus_Sig9/1  "<testSig_Air_bPerTAFSFinalDef>"
  BS/10 -> ToWs_Req_Bus_Sig10/1  "<testSig_Air_bPerTAFSProvDef>"
  BS/11 -> ToWs_Req_Bus_Sig11/1  "<testSig_Air_facPerCorTAFS>"
  BS/12 -> ToWs_Req_Bus_Sig12/1  "<testSig_Air_bDtyCycHiDebTAFS_DSM>"
  BS/13 -> ToWs_Req_Bus_Sig13/1  "<testSig_Air_bDtyCycLoDebTAFS_DSM>"
  BS/14 -> ToWs_Req_Bus_Sig14/1  "<testSig_Air_bPerHiDebTAFS_DSM>"
  BS/15 -> ToWs_Req_Bus_Sig15/1  "<testSig_Air_bPerLoDebTAFS_DSM>"
  BS/16 -> ToWs_Req_Bus_Sig16/1  "<testSig_Air_bVoltTAFSFinalDef>"
  BS/17 -> ToWs_Req_Bus_Sig17/1  "<testSig_Air_bVoltTAFSProvDef>"
  BS/18 -> ToWs_Req_Bus_Sig18/1  "<testSig_Air_bVoltHiDebTAFS_DSM>"
  BS/19 -> ToWs_Req_Bus_Sig19/1  "<testSig_Air_bVoltLoDebTAFS_DSM>"
  sig_Result_Bus/1 -> BS_Result/1, specifyOutputs/2(sig_Result_Bus)
  BS_Result/1 -> ToWs_Result_Bus_Sig1/1  "<Air_tSensTAFS>"
  BS_Result/2 -> ToWs_Result_Bus_Sig2/1  "<Air_bDtyCycTAFSFinalDef>"
  BS_Result/3 -> ToWs_Result_Bus_Sig3/1  "<Air_bDtyCycTAFSProvDef>"
  BS_Result/4 -> ToWs_Result_Bus_Sig4/1  "<Air_bPerTAFSFinalDef>"
  BS_Result/5 -> ToWs_Result_Bus_Sig5/1  "<Air_bPerTAFSProvDef>"
  BS_Result/6 -> ToWs_Result_Bus_Sig6/1  "<Air_facPerCorTAFS>"
  BS_Result/7 -> ToWs_Result_Bus_Sig7/1  "<Air_bDtyCycHiDebTAFS_DSM>"
  BS_Result/8 -> ToWs_Result_Bus_Sig8/1  "<Air_bDtyCycLoDebTAFS_DSM>"
  BS_Result/9 -> ToWs_Result_Bus_Sig9/1  "<Air_bPerHiDebTAFS_DSM>"
  BS_Result/10 -> ToWs_Result_Bus_Sig10/1  "<Air_bPerLoDebTAFS_DSM>"
  BS_Result/11 -> ToWs_Result_Bus_Sig11/1  "<Air_bVoltTAFSFinalDef>"
  BS_Result/12 -> ToWs_Result_Bus_Sig12/1  "<Air_bVoltTAFSProvDef>"
  BS_Result/13 -> ToWs_Result_Bus_Sig13/1  "<Air_bVoltHiDebTAFS_DSM>"
  BS_Result/14 -> ToWs_Result_Bus_Sig14/1  "<Air_bVoltLoDebTAFS_DSM>"
  specifyOutputs/1(result) -> result/1

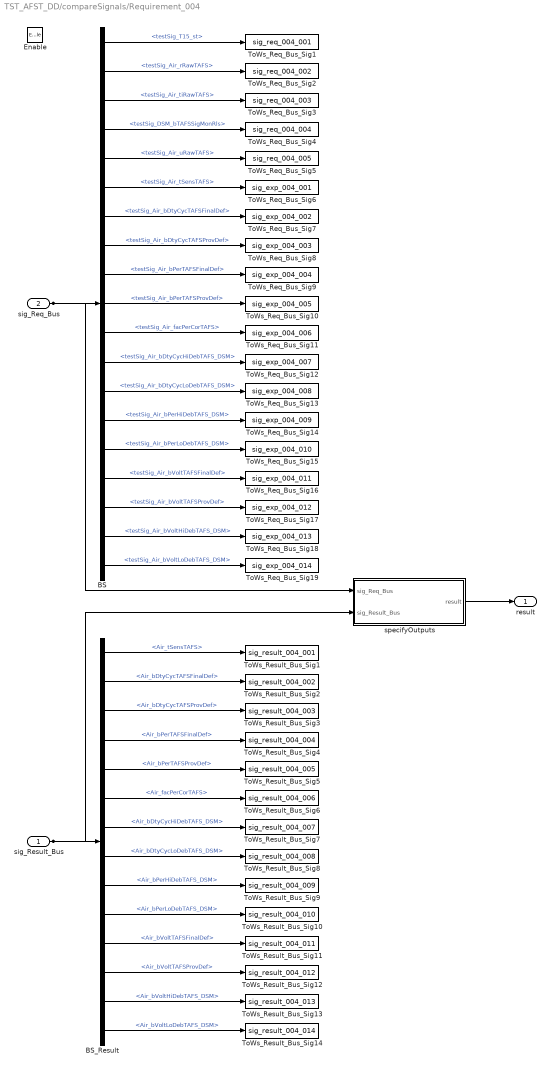
== system TST_AFST_DD/compareSignals/Requirement_004 ==
  sig_Result_Bus : Inport
  sig_Req_Bus : Inport  Port=2
  Enable : EnablePort
  BS : BusSelector  OutputSignals=testSig_T15_st,testSig_Air_rRawTAFS,testSig_Air_tiRawTAFS,testSig_DSM_bTAFSSigMonRls,testSig_Air_uRawTAFS,testSig_Air_tSensTAFS,testSig_Air_bDtyCycTAFSFinalDef,testSig_Air_bDtyCycTAFSProvDef,testSig_Air_bPerTAFSFinalDef,testSig_Air_bPerTAFSProvDef,testSig_Air_facPerCorTAFS,testSig_Air_bDtyCycHiDebTAFS_DSM,testSig_Air_bDtyCycLoDebTAFS_DSM,testSig_Air_bPerHiDebTAFS_DSM,testSig_Air_bPerLoDebTAFS_DSM,testSig_Air_bVoltTAFSFinalDef,testSig_Air_bVoltTAFSProvDef,testSig_Air_bVoltHiDebTAFS_DSM,testSig_Air_bVoltLoDebTAFS_DSM
  BS_Result : BusSelector  OutputSignals=Air_tSensTAFS,Air_bDtyCycTAFSFinalDef,Air_bDtyCycTAFSProvDef,Air_bPerTAFSFinalDef,Air_bPerTAFSProvDef,Air_facPerCorTAFS,Air_bDtyCycHiDebTAFS_DSM,Air_bDtyCycLoDebTAFS_DSM,Air_bPerHiDebTAFS_DSM,Air_bPerLoDebTAFS_DSM,Air_bVoltTAFSFinalDef,Air_bVoltTAFSProvDef,Air_bVoltHiDebTAFS_DSM,Air_bVoltLoDebTAFS_DSM
  ToWs_Req_Bus_Sig1 : ToWorkspace  VariableName=sig_req_004_001  SaveFormat=Structure With Time
  ToWs_Req_Bus_Sig10 : ToWorkspace  VariableName=sig_exp_004_005  SaveFormat=Structure With Time
  ToWs_Req_Bus_Sig11 : ToWorkspace  VariableName=sig_exp_004_006  SaveFormat=Structure With Time
  ToWs_Req_Bus_Sig12 : ToWorkspace  VariableName=sig_exp_004_007  SaveFormat=Structure With Time
  ToWs_Req_Bus_Sig13 : ToWorkspace  VariableName=sig_exp_004_008  SaveFormat=Structure With Time
  ToWs_Req_Bus_Sig14 : ToWorkspace  VariableName=sig_exp_004_009  SaveFormat=Structure With Time
  ToWs_Req_Bus_Sig15 : ToWorkspace  VariableName=sig_exp_004_010  SaveFormat=Structure With Time
  ToWs_Req_Bus_Sig16 : ToWorkspace  VariableName=sig_exp_004_011  SaveFormat=Structure With Time
  ToWs_Req_Bus_Sig17 : ToWorkspace  VariableName=sig_exp_004_012  SaveFormat=Structure With Time
  ToWs_Req_Bus_Sig18 : ToWorkspace  VariableName=sig_exp_004_013  SaveFormat=Structure With Time
  ToWs_Req_Bus_Sig19 : ToWorkspace  VariableName=sig_exp_004_014  SaveFormat=Structure With Time
  ToWs_Req_Bus_Sig2 : ToWorkspace  VariableName=sig_req_004_002  SaveFormat=Structure With Time
  ToWs_Req_Bus_Sig3 : ToWorkspace  VariableName=sig_req_004_003  SaveFormat=Structure With Time
  ToWs_Req_Bus_Sig4 : ToWorkspace  VariableName=sig_req_004_004  SaveFormat=Structure With Time
  ToWs_Req_Bus_Sig5 : ToWorkspace  VariableName=sig_req_004_005  SaveFormat=Structure With Time
  ToWs_Req_Bus_Sig6 : ToWorkspace  VariableName=sig_exp_004_001  SaveFormat=Structure With Time
  ToWs_Req_Bus_Sig7 : ToWorkspace  VariableName=sig_exp_004_002  SaveFormat=Structure With Time
  ToWs_Req_Bus_Sig8 : ToWorkspace  VariableName=sig_exp_004_003  SaveFormat=Structure With Time
  ToWs_Req_Bus_Sig9 : ToWorkspace  VariableName=sig_exp_004_004  SaveFormat=Structure With Time
  ToWs_Result_Bus_Sig1 : ToWorkspace  VariableName=sig_result_004_001  SaveFormat=Structure With Time
  ToWs_Result_Bus_Sig10 : ToWorkspace  VariableName=sig_result_004_010  SaveFormat=Structure With Time
  ToWs_Result_Bus_Sig11 : ToWorkspace  VariableName=sig_result_004_011  SaveFormat=Structure With Time
  ToWs_Result_Bus_Sig12 : ToWorkspace  VariableName=sig_result_004_012  SaveFormat=Structure With Time
  ToWs_Result_Bus_Sig13 : ToWorkspace  VariableName=sig_result_004_013  SaveFormat=Structure With Time
  ToWs_Result_Bus_Sig14 : ToWorkspace  VariableName=sig_result_004_014  SaveFormat=Structure With Time
  ToWs_Result_Bus_Sig2 : ToWorkspace  VariableName=sig_result_004_002  SaveFormat=Structure With Time
  ToWs_Result_Bus_Sig3 : ToWorkspace  VariableName=sig_result_004_003  SaveFormat=Structure With Time
  ToWs_Result_Bus_Sig4 : ToWorkspace  VariableName=sig_result_004_004  SaveFormat=Structure With Time
  ToWs_Result_Bus_Sig5 : ToWorkspace  VariableName=sig_result_004_005  SaveFormat=Structure With Time
  ToWs_Result_Bus_Sig6 : ToWorkspace  VariableName=sig_result_004_006  SaveFormat=Structure With Time
  ToWs_Result_Bus_Sig7 : ToWorkspace  VariableName=sig_result_004_007  SaveFormat=Structure With Time
  ToWs_Result_Bus_Sig8 : ToWorkspace  VariableName=sig_result_004_008  SaveFormat=Structure With Time
  ToWs_Result_Bus_Sig9 : ToWorkspace  VariableName=sig_result_004_009  SaveFormat=Structure With Time
  specifyOutputs : Subsystem
  result : Outport
  wires:
  sig_Req_Bus/1 -> BS/1, specifyOutputs/1(sig_Req_Bus)
  BS/1 -> ToWs_Req_Bus_Sig1/1  "<testSig_T15_st>"
  BS/2 -> ToWs_Req_Bus_Sig2/1  "<testSig_Air_rRawTAFS>"
  BS/3 -> ToWs_Req_Bus_Sig3/1  "<testSig_Air_tiRawTAFS>"
  BS/4 -> ToWs_Req_Bus_Sig4/1  "<testSig_DSM_bTAFSSigMonRls>"
  BS/5 -> ToWs_Req_Bus_Sig5/1  "<testSig_Air_uRawTAFS>"
  BS/6 -> ToWs_Req_Bus_Sig6/1  "<testSig_Air_tSensTAFS>"
  BS/7 -> ToWs_Req_Bus_Sig7/1  "<testSig_Air_bDtyCycTAFSFinalDef>"
  BS/8 -> ToWs_Req_Bus_Sig8/1  "<testSig_Air_bDtyCycTAFSProvDef>"
  BS/9 -> ToWs_Req_Bus_Sig9/1  "<testSig_Air_bPerTAFSFinalDef>"
  BS/10 -> ToWs_Req_Bus_Sig10/1  "<testSig_Air_bPerTAFSProvDef>"
  BS/11 -> ToWs_Req_Bus_Sig11/1  "<testSig_Air_facPerCorTAFS>"
  BS/12 -> ToWs_Req_Bus_Sig12/1  "<testSig_Air_bDtyCycHiDebTAFS_DSM>"
  BS/13 -> ToWs_Req_Bus_Sig13/1  "<testSig_Air_bDtyCycLoDebTAFS_DSM>"
  BS/14 -> ToWs_Req_Bus_Sig14/1  "<testSig_Air_bPerHiDebTAFS_DSM>"
  BS/15 -> ToWs_Req_Bus_Sig15/1  "<testSig_Air_bPerLoDebTAFS_DSM>"
  BS/16 -> ToWs_Req_Bus_Sig16/1  "<testSig_Air_bVoltTAFSFinalDef>"
  BS/17 -> ToWs_Req_Bus_Sig17/1  "<testSig_Air_bVoltTAFSProvDef>"
  BS/18 -> ToWs_Req_Bus_Sig18/1  "<testSig_Air_bVoltHiDebTAFS_DSM>"
  BS/19 -> ToWs_Req_Bus_Sig19/1  "<testSig_Air_bVoltLoDebTAFS_DSM>"
  sig_Result_Bus/1 -> BS_Result/1, specifyOutputs/2(sig_Result_Bus)
  BS_Result/1 -> ToWs_Result_Bus_Sig1/1  "<Air_tSensTAFS>"
  BS_Result/2 -> ToWs_Result_Bus_Sig2/1  "<Air_bDtyCycTAFSFinalDef>"
  BS_Result/3 -> ToWs_Result_Bus_Sig3/1  "<Air_bDtyCycTAFSProvDef>"
  BS_Result/4 -> ToWs_Result_Bus_Sig4/1  "<Air_bPerTAFSFinalDef>"
  BS_Result/5 -> ToWs_Result_Bus_Sig5/1  "<Air_bPerTAFSProvDef>"
  BS_Result/6 -> ToWs_Result_Bus_Sig6/1  "<Air_facPerCorTAFS>"
  BS_Result/7 -> ToWs_Result_Bus_Sig7/1  "<Air_bDtyCycHiDebTAFS_DSM>"
  BS_Result/8 -> ToWs_Result_Bus_Sig8/1  "<Air_bDtyCycLoDebTAFS_DSM>"
  BS_Result/9 -> ToWs_Result_Bus_Sig9/1  "<Air_bPerHiDebTAFS_DSM>"
  BS_Result/10 -> ToWs_Result_Bus_Sig10/1  "<Air_bPerLoDebTAFS_DSM>"
  BS_Result/11 -> ToWs_Result_Bus_Sig11/1  "<Air_bVoltTAFSFinalDef>"
  BS_Result/12 -> ToWs_Result_Bus_Sig12/1  "<Air_bVoltTAFSProvDef>"
  BS_Result/13 -> ToWs_Result_Bus_Sig13/1  "<Air_bVoltHiDebTAFS_DSM>"
  BS_Result/14 -> ToWs_Result_Bus_Sig14/1  "<Air_bVoltLoDebTAFS_DSM>"
  specifyOutputs/1(result) -> result/1

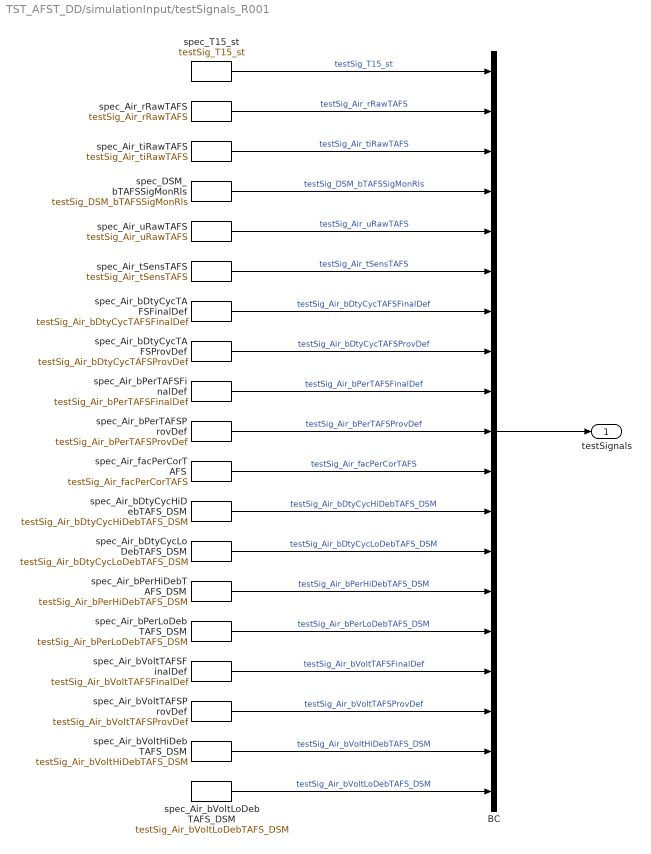
== system TST_AFST_DD/simulationInput/testSignals_R001 ==
  BC : BusCreator  Inputs=19
  spec_Air_bDtyCycHiDebTAFS_DSM : FromWorkspace  VariableName=testSig_Air_bDtyCycHiDebTAFS_DSM  Interpolate=off  OutputAfterFinalValue=Holding final value
  spec_Air_bDtyCycLoDebTAFS_DSM : FromWorkspace  VariableName=testSig_Air_bDtyCycLoDebTAFS_DSM  Interpolate=off  OutputAfterFinalValue=Holding final value
  spec_Air_bDtyCycTAFSFinalDef : FromWorkspace  VariableName=testSig_Air_bDtyCycTAFSFinalDef  Interpolate=off  OutputAfterFinalValue=Holding final value
  spec_Air_bDtyCycTAFSProvDef : FromWorkspace  VariableName=testSig_Air_bDtyCycTAFSProvDef  Interpolate=off  OutputAfterFinalValue=Holding final value
  spec_Air_bPerHiDebTAFS_DSM : FromWorkspace  VariableName=testSig_Air_bPerHiDebTAFS_DSM  Interpolate=off  OutputAfterFinalValue=Holding final value
  spec_Air_bPerLoDebTAFS_DSM : FromWorkspace  VariableName=testSig_Air_bPerLoDebTAFS_DSM  Interpolate=off  OutputAfterFinalValue=Holding final value
  spec_Air_bPerTAFSFinalDef : FromWorkspace  VariableName=testSig_Air_bPerTAFSFinalDef  Interpolate=off  OutputAfterFinalValue=Holding final value
  spec_Air_bPerTAFSProvDef : FromWorkspace  VariableName=testSig_Air_bPerTAFSProvDef  Interpolate=off  OutputAfterFinalValue=Holding final value
  spec_Air_bVoltHiDebTAFS_DSM : FromWorkspace  VariableName=testSig_Air_bVoltHiDebTAFS_DSM  Interpolate=off  OutputAfterFinalValue=Holding final value
  spec_Air_bVoltLoDebTAFS_DSM : FromWorkspace  VariableName=testSig_Air_bVoltLoDebTAFS_DSM  Interpolate=off  OutputAfterFinalValue=Holding final value
  spec_Air_bVoltTAFSFinalDef : FromWorkspace  VariableName=testSig_Air_bVoltTAFSFinalDef  Interpolate=off  OutputAfterFinalValue=Holding final value
  spec_Air_bVoltTAFSProvDef : FromWorkspace  VariableName=testSig_Air_bVoltTAFSProvDef  Interpolate=off  OutputAfterFinalValue=Holding final value
  spec_Air_facPerCorTAFS : FromWorkspace  VariableName=testSig_Air_facPerCorTAFS  Interpolate=off  OutputAfterFinalValue=Holding final value
  spec_Air_rRawTAFS : FromWorkspace  VariableName=testSig_Air_rRawTAFS  Interpolate=off  OutputAfterFinalValue=Holding final value
  spec_Air_tSensTAFS : FromWorkspace  VariableName=testSig_Air_tSensTAFS  Interpolate=off  OutputAfterFinalValue=Holding final value
  spec_Air_tiRawTAFS : FromWorkspace  VariableName=testSig_Air_tiRawTAFS  Interpolate=off  OutputAfterFinalValue=Holding final value
  spec_Air_uRawTAFS : FromWorkspace  VariableName=testSig_Air_uRawTAFS  Interpolate=off  OutputAfterFinalValue=Holding final value
  spec_DSM_bTAFSSigMonRls : FromWorkspace  VariableName=testSig_DSM_bTAFSSigMonRls  Interpolate=off  OutputAfterFinalValue=Holding final value
  spec_T15_st : FromWorkspace  VariableName=testSig_T15_st  Interpolate=off  OutputAfterFinalValue=Holding final value
  testSignals : Outport
  wires:
  BC/1 -> testSignals/1
  spec_T15_st/1 -> BC/1  "testSig_T15_st"
  spec_Air_rRawTAFS/1 -> BC/2  "testSig_Air_rRawTAFS"
  spec_Air_tiRawTAFS/1 -> BC/3  "testSig_Air_tiRawTAFS"
  spec_DSM_bTAFSSigMonRls/1 -> BC/4  "testSig_DSM_bTAFSSigMonRls"
  spec_Air_uRawTAFS/1 -> BC/5  "testSig_Air_uRawTAFS"
  spec_Air_tSensTAFS/1 -> BC/6  "testSig_Air_tSensTAFS"
  spec_Air_bDtyCycTAFSFinalDef/1 -> BC/7  "testSig_Air_bDtyCycTAFSFinalDef"
  spec_Air_bDtyCycTAFSProvDef/1 -> BC/8  "testSig_Air_bDtyCycTAFSProvDef"
  spec_Air_bPerTAFSFinalDef/1 -> BC/9  "testSig_Air_bPerTAFSFinalDef"
  spec_Air_bPerTAFSProvDef/1 -> BC/10  "testSig_Air_bPerTAFSProvDef"
  spec_Air_facPerCorTAFS/1 -> BC/11  "testSig_Air_facPerCorTAFS"
  spec_Air_bDtyCycHiDebTAFS_DSM/1 -> BC/12  "testSig_Air_bDtyCycHiDebTAFS_DSM"
  spec_Air_bDtyCycLoDebTAFS_DSM/1 -> BC/13  "testSig_Air_bDtyCycLoDebTAFS_DSM"
  spec_Air_bPerHiDebTAFS_DSM/1 -> BC/14  "testSig_Air_bPerHiDebTAFS_DSM"
  spec_Air_bPerLoDebTAFS_DSM/1 -> BC/15  "testSig_Air_bPerLoDebTAFS_DSM"
  spec_Air_bVoltTAFSFinalDef/1 -> BC/16  "testSig_Air_bVoltTAFSFinalDef"
  spec_Air_bVoltTAFSProvDef/1 -> BC/17  "testSig_Air_bVoltTAFSProvDef"
  spec_Air_bVoltHiDebTAFS_DSM/1 -> BC/18  "testSig_Air_bVoltHiDebTAFS_DSM"
  spec_Air_bVoltLoDebTAFS_DSM/1 -> BC/19  "testSig_Air_bVoltLoDebTAFS_DSM"

== system TST_AFST_DD/simulationInput/testSignals_R002 ==
  BC : BusCreator  Inputs=19
  spec_Air_bDtyCycHiDebTAFS_DSM : FromWorkspace  VariableName=testSig_Air_bDtyCycHiDebTAFS_DSM  Interpolate=off  OutputAfterFinalValue=Holding final value
  spec_Air_bDtyCycLoDebTAFS_DSM : FromWorkspace  VariableName=testSig_Air_bDtyCycLoDebTAFS_DSM  Interpolate=off  OutputAfterFinalValue=Holding final value
  spec_Air_bDtyCycTAFSFinalDef : FromWorkspace  VariableName=testSig_Air_bDtyCycTAFSFinalDef  Interpolate=off  OutputAfterFinalValue=Holding final value
  spec_Air_bDtyCycTAFSProvDef : FromWorkspace  VariableName=testSig_Air_bDtyCycTAFSProvDef  Interpolate=off  OutputAfterFinalValue=Holding final value
  spec_Air_bPerHiDebTAFS_DSM : FromWorkspace  VariableName=testSig_Air_bPerHiDebTAFS_DSM  Interpolate=off  OutputAfterFinalValue=Holding final value
  spec_Air_bPerLoDebTAFS_DSM : FromWorkspace  VariableName=testSig_Air_bPerLoDebTAFS_DSM  Interpolate=off  OutputAfterFinalValue=Holding final value
  spec_Air_bPerTAFSFinalDef : FromWorkspace  VariableName=testSig_Air_bPerTAFSFinalDef  Interpolate=off  OutputAfterFinalValue=Holding final value
  spec_Air_bPerTAFSProvDef : FromWorkspace  VariableName=testSig_Air_bPerTAFSProvDef  Interpolate=off  OutputAfterFinalValue=Holding final value
  spec_Air_bVoltHiDebTAFS_DSM : FromWorkspace  VariableName=testSig_Air_bVoltHiDebTAFS_DSM  Interpolate=off  OutputAfterFinalValue=Holding final value
  spec_Air_bVoltLoDebTAFS_DSM : FromWorkspace  VariableName=testSig_Air_bVoltLoDebTAFS_DSM  Interpolate=off  OutputAfterFinalValue=Holding final value
  spec_Air_bVoltTAFSFinalDef : FromWorkspace  VariableName=testSig_Air_bVoltTAFSFinalDef  Interpolate=off  OutputAfterFinalValue=Holding final value
  spec_Air_bVoltTAFSProvDef : FromWorkspace  VariableName=testSig_Air_bVoltTAFSProvDef  Interpolate=off  OutputAfterFinalValue=Holding final value
  spec_Air_facPerCorTAFS : FromWorkspace  VariableName=testSig_Air_facPerCorTAFS  Interpolate=off  OutputAfterFinalValue=Holding final value
  spec_Air_rRawTAFS : FromWorkspace  VariableName=testSig_Air_rRawTAFS  Interpolate=off  OutputAfterFinalValue=Holding final value
  spec_Air_tSensTAFS : FromWorkspace  VariableName=testSig_Air_tSensTAFS  Interpolate=off  OutputAfterFinalValue=Holding final value
  spec_Air_tiRawTAFS : FromWorkspace  VariableName=testSig_Air_tiRawTAFS  Interpolate=off  OutputAfterFinalValue=Holding final value
  spec_Air_uRawTAFS : FromWorkspace  VariableName=testSig_Air_uRawTAFS  Interpolate=off  OutputAfterFinalValue=Holding final value
  spec_DSM_bTAFSSigMonRls : FromWorkspace  VariableName=testSig_DSM_bTAFSSigMonRls  Interpolate=off  OutputAfterFinalValue=Holding final value
  spec_T15_st : FromWorkspace  VariableName=testSig_T15_st  Interpolate=off  OutputAfterFinalValue=Holding final value
  testSignals : Outport
  wires:
  BC/1 -> testSignals/1
  spec_T15_st/1 -> BC/1  "testSig_T15_st"
  spec_Air_rRawTAFS/1 -> BC/2  "testSig_Air_rRawTAFS"
  spec_Air_tiRawTAFS/1 -> BC/3  "testSig_Air_tiRawTAFS"
  spec_DSM_bTAFSSigMonRls/1 -> BC/4  "testSig_DSM_bTAFSSigMonRls"
  spec_Air_uRawTAFS/1 -> BC/5  "testSig_Air_uRawTAFS"
  spec_Air_tSensTAFS/1 -> BC/6  "testSig_Air_tSensTAFS"
  spec_Air_bDtyCycTAFSFinalDef/1 -> BC/7  "testSig_Air_bDtyCycTAFSFinalDef"
  spec_Air_bDtyCycTAFSProvDef/1 -> BC/8  "testSig_Air_bDtyCycTAFSProvDef"
  spec_Air_bPerTAFSFinalDef/1 -> BC/9  "testSig_Air_bPerTAFSFinalDef"
  spec_Air_bPerTAFSProvDef/1 -> BC/10  "testSig_Air_bPerTAFSProvDef"
  spec_Air_facPerCorTAFS/1 -> BC/11  "testSig_Air_facPerCorTAFS"
  spec_Air_bDtyCycHiDebTAFS_DSM/1 -> BC/12  "testSig_Air_bDtyCycHiDebTAFS_DSM"
  spec_Air_bDtyCycLoDebTAFS_DSM/1 -> BC/13  "testSig_Air_bDtyCycLoDebTAFS_DSM"
  spec_Air_bPerHiDebTAFS_DSM/1 -> BC/14  "testSig_Air_bPerHiDebTAFS_DSM"
  spec_Air_bPerLoDebTAFS_DSM/1 -> BC/15  "testSig_Air_bPerLoDebTAFS_DSM"
  spec_Air_bVoltTAFSFinalDef/1 -> BC/16  "testSig_Air_bVoltTAFSFinalDef"
  spec_Air_bVoltTAFSProvDef/1 -> BC/17  "testSig_Air_bVoltTAFSProvDef"
  spec_Air_bVoltHiDebTAFS_DSM/1 -> BC/18  "testSig_Air_bVoltHiDebTAFS_DSM"
  spec_Air_bVoltLoDebTAFS_DSM/1 -> BC/19  "testSig_Air_bVoltLoDebTAFS_DSM"

== system TST_AFST_DD/simulationInput/testSignals_R003 ==
  BC : BusCreator  Inputs=19
  spec_Air_bDtyCycHiDebTAFS_DSM : FromWorkspace  VariableName=testSig_Air_bDtyCycHiDebTAFS_DSM  Interpolate=off  OutputAfterFinalValue=Holding final value
  spec_Air_bDtyCycLoDebTAFS_DSM : FromWorkspace  VariableName=testSig_Air_bDtyCycLoDebTAFS_DSM  Interpolate=off  OutputAfterFinalValue=Holding final value
  spec_Air_bDtyCycTAFSFinalDef : FromWorkspace  VariableName=testSig_Air_bDtyCycTAFSFinalDef  Interpolate=off  OutputAfterFinalValue=Holding final value
  spec_Air_bDtyCycTAFSProvDef : FromWorkspace  VariableName=testSig_Air_bDtyCycTAFSProvDef  Interpolate=off  OutputAfterFinalValue=Holding final value
  spec_Air_bPerHiDebTAFS_DSM : FromWorkspace  VariableName=testSig_Air_bPerHiDebTAFS_DSM  Interpolate=off  OutputAfterFinalValue=Holding final value
  spec_Air_bPerLoDebTAFS_DSM : FromWorkspace  VariableName=testSig_Air_bPerLoDebTAFS_DSM  Interpolate=off  OutputAfterFinalValue=Holding final value
  spec_Air_bPerTAFSFinalDef : FromWorkspace  VariableName=testSig_Air_bPerTAFSFinalDef  Interpolate=off  OutputAfterFinalValue=Holding final value
  spec_Air_bPerTAFSProvDef : FromWorkspace  VariableName=testSig_Air_bPerTAFSProvDef  Interpolate=off  OutputAfterFinalValue=Holding final value
  spec_Air_bVoltHiDebTAFS_DSM : FromWorkspace  VariableName=testSig_Air_bVoltHiDebTAFS_DSM  Interpolate=off  OutputAfterFinalValue=Holding final value
  spec_Air_bVoltLoDebTAFS_DSM : FromWorkspace  VariableName=testSig_Air_bVoltLoDebTAFS_DSM  Interpolate=off  OutputAfterFinalValue=Holding final value
  spec_Air_bVoltTAFSFinalDef : FromWorkspace  VariableName=testSig_Air_bVoltTAFSFinalDef  Interpolate=off  OutputAfterFinalValue=Holding final value
  spec_Air_bVoltTAFSProvDef : FromWorkspace  VariableName=testSig_Air_bVoltTAFSProvDef  Interpolate=off  OutputAfterFinalValue=Holding final value
  spec_Air_facPerCorTAFS : FromWorkspace  VariableName=testSig_Air_facPerCorTAFS  Interpolate=off  OutputAfterFinalValue=Holding final value
  spec_Air_rRawTAFS : FromWorkspace  VariableName=testSig_Air_rRawTAFS  Interpolate=off  OutputAfterFinalValue=Holding final value
  spec_Air_tSensTAFS : FromWorkspace  VariableName=testSig_Air_tSensTAFS  Interpolate=off  OutputAfterFinalValue=Holding final value
  spec_Air_tiRawTAFS : FromWorkspace  VariableName=testSig_Air_tiRawTAFS  Interpolate=off  OutputAfterFinalValue=Holding final value
  spec_Air_uRawTAFS : FromWorkspace  VariableName=testSig_Air_uRawTAFS  Interpolate=off  OutputAfterFinalValue=Holding final value
  spec_DSM_bTAFSSigMonRls : FromWorkspace  VariableName=testSig_DSM_bTAFSSigMonRls  Interpolate=off  OutputAfterFinalValue=Holding final value
  spec_T15_st : FromWorkspace  VariableName=testSig_T15_st  Interpolate=off  OutputAfterFinalValue=Holding final value
  testSignals : Outport
  wires:
  BC/1 -> testSignals/1
  spec_T15_st/1 -> BC/1  "testSig_T15_st"
  spec_Air_rRawTAFS/1 -> BC/2  "testSig_Air_rRawTAFS"
  spec_Air_tiRawTAFS/1 -> BC/3  "testSig_Air_tiRawTAFS"
  spec_DSM_bTAFSSigMonRls/1 -> BC/4  "testSig_DSM_bTAFSSigMonRls"
  spec_Air_uRawTAFS/1 -> BC/5  "testSig_Air_uRawTAFS"
  spec_Air_tSensTAFS/1 -> BC/6  "testSig_Air_tSensTAFS"
  spec_Air_bDtyCycTAFSFinalDef/1 -> BC/7  "testSig_Air_bDtyCycTAFSFinalDef"
  spec_Air_bDtyCycTAFSProvDef/1 -> BC/8  "testSig_Air_bDtyCycTAFSProvDef"
  spec_Air_bPerTAFSFinalDef/1 -> BC/9  "testSig_Air_bPerTAFSFinalDef"
  spec_Air_bPerTAFSProvDef/1 -> BC/10  "testSig_Air_bPerTAFSProvDef"
  spec_Air_facPerCorTAFS/1 -> BC/11  "testSig_Air_facPerCorTAFS"
  spec_Air_bDtyCycHiDebTAFS_DSM/1 -> BC/12  "testSig_Air_bDtyCycHiDebTAFS_DSM"
  spec_Air_bDtyCycLoDebTAFS_DSM/1 -> BC/13  "testSig_Air_bDtyCycLoDebTAFS_DSM"
  spec_Air_bPerHiDebTAFS_DSM/1 -> BC/14  "testSig_Air_bPerHiDebTAFS_DSM"
  spec_Air_bPerLoDebTAFS_DSM/1 -> BC/15  "testSig_Air_bPerLoDebTAFS_DSM"
  spec_Air_bVoltTAFSFinalDef/1 -> BC/16  "testSig_Air_bVoltTAFSFinalDef"
  spec_Air_bVoltTAFSProvDef/1 -> BC/17  "testSig_Air_bVoltTAFSProvDef"
  spec_Air_bVoltHiDebTAFS_DSM/1 -> BC/18  "testSig_Air_bVoltHiDebTAFS_DSM"
  spec_Air_bVoltLoDebTAFS_DSM/1 -> BC/19  "testSig_Air_bVoltLoDebTAFS_DSM"
